simulink model "controlMDLV2"  (Simulink 7.9)
settings: Solver=ode45  StartTime=0.0  StopTime=inf  RelTol=1e-3
libraries: dspmtrx3 x7, simulink x7, utility x1, dspsolvers x1
settings Model: Creator=jorhabib  LastModifiedBy=jorhabib

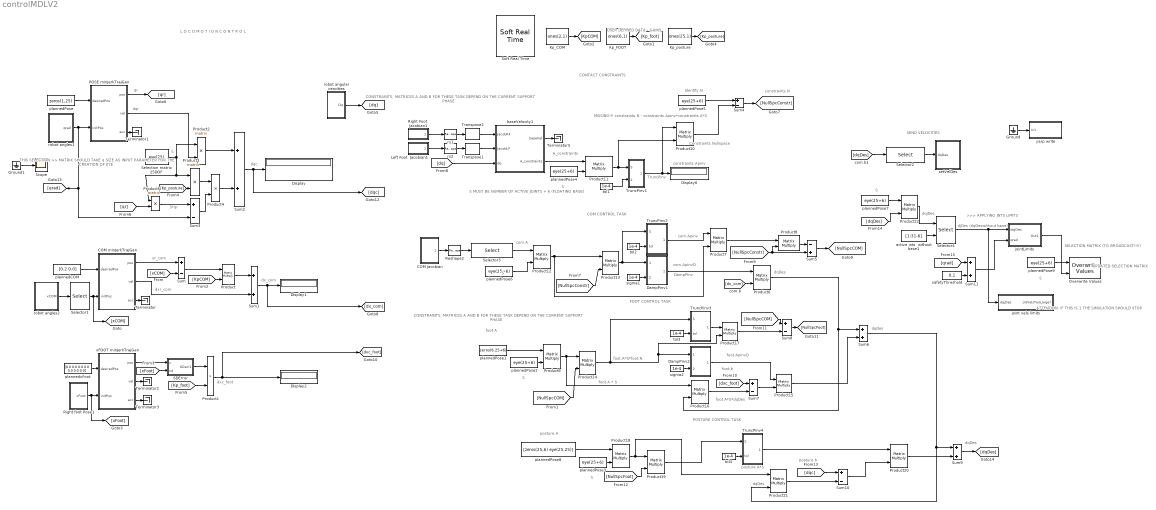
== system controlMDLV2 ==
  note: qr
  note: dqr
  note: S
  note: dqc
  note: S*qr
  note: THIS SELECTION    >>
      | MATRIX SHOULD
      | TAKE q SIZE AS
      | INPUT PARAMETER
      | FOR THE CREATION
      | OF EYE
  note: USER DEFINED DATA - GAINS
  note: xr_com
  note: dx_com
  note: dxr_com
  note: dxc_foot
  note: A_constraints
  note: S
  note: TruncPinv
  note: S MUST BE NUMBER OF
      | ACTIVE JOINTS
      | + 6 (FLOATING BASE)
  note: constraints.Apinv
  note: constraints.N
  note: Constraints
      | Nullspace
  note: MISSING!!! constraints.N - constraints.Apinv*constraints.A*S
  note: Identity.N
  note: CONTACT CONSTRAINTS
  note: CONSTRAINTS, MATRICES
      |  A AND B FOR THESE TASK DEPEND
      | ON THE CURRENT SUPPORT PHASE
  note: DampPInv
  note: com.A
  note: S
  note: com.ApinvD
  note: COM CONTROL TASK
  note: FOOT CONTROL TASK
  note: dqDes
  note: com.Apinv
  note: CONSTRAINTS, MATRICES
      |  A AND B FOR THESE TASK DEPEND
      | ON THE CURRENT SUPPORT PHASE
  note: S
  note: foot.A
  note: dqDes
  note: POSTURE CONTROL TASK
  note: posture.A
  note: S
  note: posture.A*S
  note: dqDes
  note: dqDes
  note: foot.ApinvD
  note: foot.b
  note: foot.A*S*dqDes
  note: posture.b
  note: foot.A * S
  note: foot.A*S*foot.N
  note: SEND VELOCITIES
  note: L O C O M O T I O N C O N T R O L
  note: S
  note: dqjDes
  note: >>> APPLYING JNTS LIMITS
  note: djDes
      |  (dqDeswithout base)
  note: SELECTION MATRIX
      |  (TO BROADCAST!!!!)
  note: S
  note: UPDATED
      | SELECTION
      | MATRIX
  note: ATTENTION: IF THIS IS 1
      | THE SIMULATION
      | SHOULD STOP
  6DError : Subsystem
  COM Jacobian : Subsystem
  COM minJerkTrajGen : Subsystem
  DampPinv1 : Subsystem  mask{tol=1e-4}
      mask prompts: tol "Tolerance"
  DampPinv2 : Subsystem  mask{tol=1e-4}
      mask prompts: tol "Tolerance"
  Display{,1..2,6} (4 alike) : Display
  Ground : Ground
  Ground1 : Ground
  Kp_COM : Constant  Value=ones(2,1)
  Kp_FOOT : Constant  Value=ones(6,1)
  Kp_posture : Constant  Value=ones(25,1)
  Left Foot  Jacobian1 : Subsystem
  Overwrite Values : dspmtrx3/Overwrite Values  OverWriteDiag=Submatrix  valFrom2ndIP=Second input port  ConstValue=0  RowSpan=Range of rows  RowStartMode=Index  RowStartIndex=7  RowEndMode=Last  RowEndIndex=31  ColSpan=Range of columns  ColStartMode=Index  ColStartIndex=7  ColEndMode=Last  ColEndIndex=1  DiagSpan=Range of elements  DiagStartMode=Index  DiagStartIndex=2  DiagEndMode=Index  DiagEndIndex=4
  POSE minJerkTrajGen : Subsystem
  Product{,2..3,5..22} (21 alike) : Product  Multiplication=Matrix(*)  RndMeth=Zero
  Product1 : Product  RndMeth=Zero
  Product4 : Product  RndMeth=Zero
  Reshape2 : Reshape  OutputDimensionality=Customize  OutputDimensions=[6,31]
  Right Foot  Jacobian1 : Subsystem
  Right foot Pose1 : Subsystem
  Scope : Scope
  Selection matrix 25DOF : Constant  Value=eye(25)
  Selector1 : Selector  IndexMode=Zero-based  InputPortWidth=7  IndexOptions=Index vector (dialog)  Indices=[0:1]  OutputSizes=1
  Selector2 : Selector  InputPortWidth=31  IndexOptions=Index vector (dialog)  Indices=[7:31]  OutputSizes=1
  Selector3 : Selector  NumberOfDimensions=2  IndexMode=Zero-based  InputPortWidth=7  IndexOptions=Starting index (dialog),Starting index (dialog)  Indices=0,0  OutputSizes=2,25+6
  Selector4 : Selector  InputPortWidth=31  IndexOptions=Index vector (port)  Indices=[0:1]  OutputSizes=1
  Soft Real Time : utility/Soft Real Time  x=0.050
  Sum{,3..4,7..8,10} (6 alike) : Sum  Inputs=+-
  Sum{1..2,6,9,11} (5 alike) : Sum
  Sum5 : Sum  Inputs=-+
  Terminator{,1..3,5} (5 alike) : Terminator
  Transpose1 : dspmtrx3/Transpose  Hermitian=off  overflowFlag=off
  Transpose2 : dspmtrx3/Transpose  Hermitian=off  overflowFlag=off
  TruncPinv1 : Subsystem  mask{tol=1e-4}
      mask prompts: tol "Tolerance"
  TruncPinv2 : Subsystem  mask{tol=1e-4}
      mask prompts: tol "Tolerance"
  TruncPinv3 : Subsystem  mask{tol=1e-4}
      mask prompts: tol "Tolerance"
  TruncPinv4 : Subsystem  mask{tol=1e-4}
      mask prompts: tol "Tolerance"
  active jnts  without base1 : Constant  Value=[1:31-6]
  baseVelocity1 : Subsystem
  joint vels limits : Subsystem  mask{dqMax=1.0}
      mask prompts: dqMax "Maximum joint velocity"
      mask help:
      | Type a vector with the maximum values for each joint (e.g. 150*ones(25,1) for a 25 DOF robot)
      | Same for minimum joint limits.
      mask init:
      | qMax = 150*ones(25,1)
      | qMin = -150*ones(25,1)
      | thr = 0.1
  jointLimits : Subsystem  mask{qMax=150*ones(25,1), qMin=-150*ones(25,1), thr=0.1}
      mask prompts: qMax "Maximum joint angles vector"; qMin "Minimum joint angles vector"; thr "Threshold before hitting joint limit"
      mask help:
      | Type a vector with the maximum values for each joint (e.g. 150*ones(25,1) for a 25 DOF robot)
      | Same for minimum joint limits.
      mask init:
      | qMax = 150*ones(25,1)
      | qMin = -150*ones(25,1)
      | thr = 0.1
  plannedCOM : Constant  Value=[0.2 0.0]
  plannedPose : Constant  Value=zeros(1,25)
  plannedPose1 : Constant  Value=zeros(6,25+6)
  plannedPose{2..7,9} (7 alike) : Constant  Value=eye(25+6)
  plannedPose8 : Constant  Value=[zeros(25,6) eye(25,25)]
  plannedxFoot : Constant  Value=[0.0 0.0 0.0 0.0 0.0 0.0 0.0]
  robot angles1 : Subsystem
  robot angles2 : Subsystem
  robot angular veocities : Subsystem
  rs1 : Reshape  OutputDimensionality=Customize  OutputDimensions=[31,6]
  rs2 : Reshape  OutputDimensionality=Customize  OutputDimensions=[31,6]
  safetyThreshold : Constant  Value=0.1
  setVelDes : Subsystem
  sigma1 : Constant  Value=1e-4
  sigma2 : Constant  Value=1e-4
  tol{1..4} (4 alike) : Constant  Value=1e-4
  xFOOT minJerkTrajGen : Subsystem
  yarp write : Subsystem  mask{port_name='/ywrite:o'}
      mask prompts: port_name "Specify port name starting with "/" e.g. '/port/input:i'"
  wires:
  robot angles1/1(qrad) -> [qrad], Sum3/2, POSE minJerkTrajGen/2(initPos)
  plannedPose/1 -> POSE minJerkTrajGen/1(desiredPos)
  Selection matrix 25DOF/1 -> Product2/1, Product5/1, Product3/1
  Product2/1 -> Sum2/1
  [Kp_posture] -> Product3/2
  Product3/1 -> Product4/1
  Sum3/1 -> Product4/2
  Product4/1 -> Sum2/2
  Sum2/1 -> [dqc], Display/1
  Product5/1 -> Sum3/1
  POSE minJerkTrajGen/3(acc) -> Terminator1/1
  POSE minJerkTrajGen/1(pos) -> [qr]
  [qr] -> Product5/2
  POSE minJerkTrajGen/2(vel) -> Product2/2
  Kp_COM/1 -> [KpCOM]
  Kp_FOOT/1 -> [Kp_foot]
  Kp_posture/1 -> [Kp_posture]
  plannedCOM/1 -> COM minJerkTrajGen/1(desiredPos)
  COM minJerkTrajGen/1(pos) -> Sum/1
  COM minJerkTrajGen/3(acc) -> Terminator/1
  [xCOM] -> Sum/2
  Sum/1 -> Product/1
  [KpCOM] -> Product/2
  Product/1 -> Sum1/1
  COM minJerkTrajGen/2(vel) -> Sum1/2
  Sum1/1 -> [dx_com], Display1/1
  Selector1/1 -> [xCOM], COM minJerkTrajGen/2(initPos)
  robot angles2/1(xCOM) -> Selector1/1
  xFOOT minJerkTrajGen/1(pos) -> 6DError/1(x)
  Right foot Pose1/1(xFoot) -> [xFoot], xFOOT minJerkTrajGen/2(initPos)
  plannedxFoot/1 -> xFOOT minJerkTrajGen/1(desiredPos)
  [xFoot] -> 6DError/2(xd)
  [Kp_foot] -> Product1/2
  Product1/1 -> [dxc_foot], Display2/1
  6DError/1(6Derr1) -> Product1/1
  xFOOT minJerkTrajGen/3(acc) -> Terminator3/1
  xFOOT minJerkTrajGen/2(vel) -> Terminator2/1
  robot angular veocities/1(Dq) -> [dq]
  Right Foot  Jacobian1/1(Jacobian) -> rs1/1
  Left Foot  Jacobian1/1(Jacobian) -> rs2/1
  [dq] -> baseVelocity1/3(dq)
  baseVelocity1/2(A_constraints) -> Product11/1
  plannedPose4/1 -> Product11/2
  tol1/1 -> TruncPinv1/2(tol)
  Product11/1 -> TruncPinv1/1(S), Product10/2
  TruncPinv1/1(Tpinv) -> Display6/1, Product10/1
  baseVelocity1/1(baseVel) -> Terminator5/1
  Product10/1 -> Sum4/2
  plannedPose5/1 -> Sum4/1
  Sum4/1 -> [NullSpcConstr]
  sigma1/1 -> DampPinv1/2(sigma)
  DampPinv1/1(DPinv) -> Product6/1
  COM Jacobian/1(Jacobian) -> Reshape2/1
  Reshape2/1 -> Selector3/1
  Selector3/1 -> Product12/1
  plannedPose6/1 -> Product12/2
  Product12/1 -> Product7/2, Product13/1
  [NullSpcConstr] -> Product13/2
  Product13/1 -> DampPinv1/1(mat), TruncPinv2/1(S)
  [dx_com] -> Product6/2
  Product6/1 -> Product16/2, Sum6/1
  tol2/1 -> TruncPinv2/2(tol)
  TruncPinv2/1(Tpinv) -> Product7/1
  Product7/1 -> Product8/1
  [NullSpcConstr] -> Sum5/2, Product8/2
  Product8/1 -> Sum5/1
  Sum5/1 -> [NullSpcCOM]
  tol3/1 -> TruncPinv3/2(tol)
  sigma2/1 -> DampPinv2/2(sigma)
  plannedPose1/1 -> Product9/1
  plannedPose2/1 -> Product9/2
  Product9/1 -> Product16/1, Product14/1
  [NullSpcCOM] -> Product14/2
  Product14/1 -> Product17/2, DampPinv2/1(mat), TruncPinv3/1(S)
  [dxc_foot] -> Sum7/1
  Product16/1 -> Sum7/2
  Product15/1 -> Sum6/2
  [NullSpcCOM] -> Sum8/1
  TruncPinv3/1(Tpinv) -> Product17/1
  Product17/1 -> Sum8/2
  Sum8/1 -> [NullSpcFoot]
  tol4/1 -> TruncPinv4/2(tol)
  plannedPose3/1 -> Product18/2
  plannedPose8/1 -> Product18/1
  Product18/1 -> Product21/1, Product19/1
  [NullSpcFoot] -> Product19/2
  Product19/1 -> TruncPinv4/1(S)
  Sum6/1 -> Product21/2, Sum9/1
  TruncPinv4/1(Tpinv) -> Product20/1
  [dqc] -> Sum10/1
  Product21/1 -> Sum10/2
  Sum10/1 -> Product20/2
  Product20/1 -> Sum9/2
  DampPinv2/1(DPinv) -> Product15/1
  Sum7/1 -> Product15/2
  Sum9/1 -> [dqDes]
  rs1/1 -> Transpose2/1
  rs2/1 -> Transpose1/1
  Transpose2/1 -> baseVelocity1/1(JacobRF)
  Transpose1/1 -> baseVelocity1/2(JacobLF)
  [dqDes] -> Selector2/1
  Selector2/1 -> setVelDes/1(dqDes)
  plannedPose7/1 -> Product22/1
  [dqDes] -> Product22/2
  Product22/1 -> Selector4/1
  active jnts  without base1/1 -> Selector4/2
  Selector4/1 -> jointLimits/1(dqjDes), joint vels limits/1(dqjDes)
  Sum11/1 -> jointLimits/2(qrad)
  [qrad] -> Sum11/1
  safetyThreshold/1 -> Sum11/2
  plannedPose9/1 -> Overwrite Values/1
  jointLimits/1(Out1) -> Overwrite Values/2
  Ground/1 -> yarp write/1(In1)
  Ground1/1 -> Scope/1

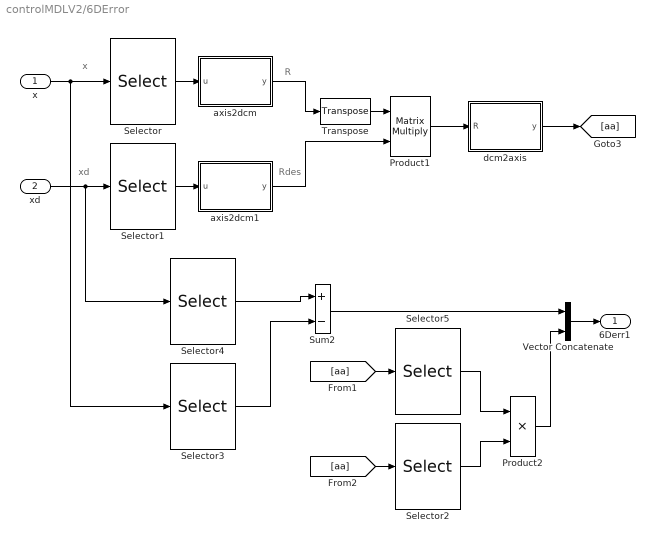
== system controlMDLV2/6DError ==
  note: xd
  note: x
  note: Rdes
  note: R
  x : Inport
  xd : Inport  Port=2
  Product1 : Product  Multiplication=Matrix(*)  RndMeth=Zero
  Product2 : Product  RndMeth=Zero
  Selector : Selector  IndexMode=Zero-based  InputPortWidth=7  IndexOptions=Index vector (dialog)  Indices=[3:6]  OutputSizes=1
  Selector1 : Selector  IndexMode=Zero-based  InputPortWidth=7  IndexOptions=Index vector (dialog)  Indices=[3:6]  OutputSizes=1
  Selector2 : Selector  IndexMode=Zero-based  InputPortWidth=4  IndexOptions=Index vector (dialog)  Indices=[0:2]  OutputSizes=1
  Selector3 : Selector  IndexMode=Zero-based  InputPortWidth=7  IndexOptions=Index vector (dialog)  Indices=[0:2]  OutputSizes=1
  Selector4 : Selector  IndexMode=Zero-based  InputPortWidth=7  IndexOptions=Index vector (dialog)  Indices=[0:2]  OutputSizes=1
  Selector5 : Selector  IndexMode=Zero-based  InputPortWidth=4  IndexOptions=Index vector (dialog)  Indices=3  OutputSizes=1
  Sum2 : Sum  Inputs=+-
  Transpose : dspmtrx3/Transpose  Hermitian=off  overflowFlag=off
  Vector Concatenate : Concatenate
  axis2dcm : MATLAB Function  TreatAsAtomicUnit=on
  axis2dcm1 : MATLAB Function  TreatAsAtomicUnit=on
  dcm2axis : MATLAB Function  TreatAsAtomicUnit=on
  6Derr1 : Outport
  wires:
  dcm2axis/1(y) -> [aa]
  Sum2/1 -> Vector Concatenate/1
  Vector Concatenate/1 -> 6Derr1/1
  [aa] -> Selector5/1
  Product2/1 -> Vector Concatenate/2
  Selector2/1 -> Product2/2
  Selector5/1 -> Product2/1
  [aa] -> Selector2/1
  Selector3/1 -> Sum2/2
  Selector4/1 -> Sum2/1
  Product1/1 -> dcm2axis/1(R)
  axis2dcm1/1(y) -> Product1/2
  axis2dcm/1(y) -> Transpose/1
  Transpose/1 -> Product1/1
  xd/1 -> Selector4/1, Selector1/1
  x/1 -> Selector3/1, Selector/1
  Selector1/1 -> axis2dcm1/1(u)
  Selector/1 -> axis2dcm/1(u)

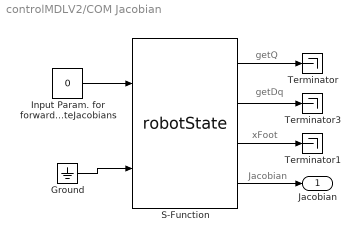
== system controlMDLV2/COM Jacobian ==
  note: getDq
  note: xFoot
  note: getQ
  note: Jacobian
  Ground : Ground
  "Input Param. for forwardKinematics and  computeJacobians " : Constant  Value=0  OutDataTypeStr=int8
  S-Function : S-Function  FunctionName=robotState  Parameters=val,robotname,localname  EnableBusSupport=off  mask{val=3, robotname='icubSim', localname='robotState'}
      mask prompts: val "Value"; robotname "Robot Name (icub - icubSim)"; localname "Module Name"
  Terminator : Terminator
  Terminator1 : Terminator
  Terminator3 : Terminator
  Jacobian : Outport
  wires:
  Ground/1 -> S-Function/2
  S-Function/2 -> Terminator3/1
  S-Function/1 -> Terminator/1
  S-Function/3 -> Terminator1/1
  "Input Param. for forwardKinematics and  computeJacobians "/1 -> S-Function/1
  S-Function/4 -> Jacobian/1

== system controlMDLV2/COM minJerkTrajGen ==
  desiredPos : Inport
  initPos : Inport  Port=2
  S-Function : S-Function  FunctionName=minJerkGenerator  Parameters=dim, rate, tt  EnableBusSupport=off  mask{dim=2, rate=10, tt=4}
      mask prompts: dim "Trajectory dimension (int)"; rate "Simulation rate (int) [ms]"; tt "Trajectory time [s]"
  pos : Outport
  vel : Outport  Port=2
  acc : Outport  Port=3
  wires:
  S-Function/2 -> vel/1
  S-Function/1 -> pos/1
  S-Function/3 -> acc/1
  initPos/1 -> S-Function/1
  desiredPos/1 -> S-Function/2

== system controlMDLV2/DampPinv1 ==
  mat : Inport
  sigma : Inport  Port=2
  Damped Pseudo Inverse : MATLAB Function  TreatAsAtomicUnit=on
  DPinv : Outport
  wires:
  sigma/1 -> Damped Pseudo Inverse/2(sigma)
  Damped Pseudo Inverse/1(DPinv) -> DPinv/1
  mat/1 -> Damped Pseudo Inverse/1(mat)

== system controlMDLV2/DampPinv2 ==
  mat : Inport
  sigma : Inport  Port=2
  Damped Pseudo Inverse : MATLAB Function  TreatAsAtomicUnit=on
  DPinv : Outport
  wires:
  mat/1 -> Damped Pseudo Inverse/1(mat)
  Damped Pseudo Inverse/1(DPinv) -> DPinv/1
  sigma/1 -> Damped Pseudo Inverse/2(sigma)

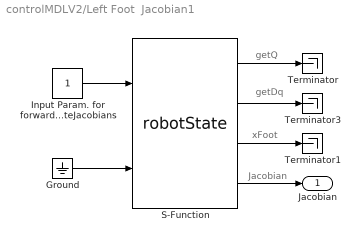
== system controlMDLV2/Left Foot  Jacobian1 ==
  note: Jacobian
  note: getQ
  note: xFoot
  note: getDq
  Ground : Ground
  "Input Param. for forwardKinematics and  computeJacobians " : Constant  OutDataTypeStr=int8
  S-Function : S-Function  FunctionName=robotState  Parameters=val,robotname,localname  EnableBusSupport=off  mask{val=3, robotname='icubSim', localname='robotState'}
      mask prompts: val "Value"; robotname "Robot Name (icub - icubSim)"; localname "Module Name"
  Terminator : Terminator
  Terminator1 : Terminator
  Terminator3 : Terminator
  Jacobian : Outport
  wires:
  S-Function/4 -> Jacobian/1
  "Input Param. for forwardKinematics and  computeJacobians "/1 -> S-Function/1
  S-Function/3 -> Terminator1/1
  S-Function/1 -> Terminator/1
  S-Function/2 -> Terminator3/1
  Ground/1 -> S-Function/2

== system controlMDLV2/POSE minJerkTrajGen ==
  desiredPos : Inport
  initPos : Inport  Port=2
  S-Function : S-Function  FunctionName=minJerkGenerator  Parameters=dim, rate, tt  EnableBusSupport=off  mask{dim=25, rate=10, tt=4}
      mask prompts: dim "Trajectory dimension (int)"; rate "Simulation rate (int) [ms]"; tt "Trajectory time [s]"
  pos : Outport
  vel : Outport  Port=2
  acc : Outport  Port=3
  wires:
  desiredPos/1 -> S-Function/2
  initPos/1 -> S-Function/1
  S-Function/3 -> acc/1
  S-Function/1 -> pos/1
  S-Function/2 -> vel/1

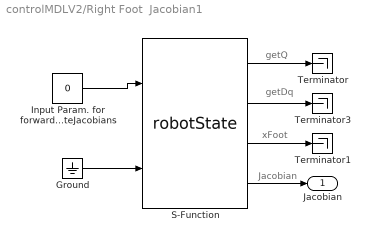
== system controlMDLV2/Right Foot  Jacobian1 ==
  note: getDq
  note: xFoot
  note: getQ
  note: Jacobian
  Ground : Ground
  "Input Param. for forwardKinematics and  computeJacobians " : Constant  Value=0  OutDataTypeStr=int8
  S-Function : S-Function  FunctionName=robotState  Parameters=val,robotname,localname  EnableBusSupport=off  mask{val=3, robotname='icubSim', localname='robotState'}
      mask prompts: val "Value"; robotname "Robot Name (icub - icubSim)"; localname "Module Name"
  Terminator : Terminator
  Terminator1 : Terminator
  Terminator3 : Terminator
  Jacobian : Outport
  wires:
  S-Function/2 -> Terminator3/1
  S-Function/1 -> Terminator/1
  S-Function/3 -> Terminator1/1
  "Input Param. for forwardKinematics and  computeJacobians "/1 -> S-Function/1
  S-Function/4 -> Jacobian/1
  Ground/1 -> S-Function/2

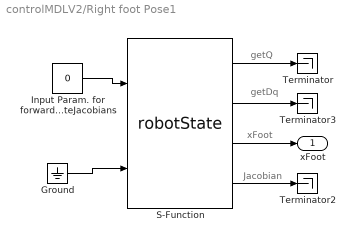
== system controlMDLV2/Right foot Pose1 ==
  note: Jacobian
  note: getQ
  note: xFoot
  note: getDq
  Ground : Ground
  "Input Param. for forwardKinematics and  computeJacobians " : Constant  Value=0  OutDataTypeStr=int8
  S-Function : S-Function  FunctionName=robotState  Parameters=val,robotname,localname  EnableBusSupport=off  mask{val=2, robotname='icubSim', localname='robotState'}
      mask prompts: val "Value"; robotname "Robot Name (icub - icubSim)"; localname "Module Name"
  Terminator : Terminator
  Terminator2 : Terminator
  Terminator3 : Terminator
  xFoot : Outport
  wires:
  Ground/1 -> S-Function/2
  S-Function/4 -> Terminator2/1
  "Input Param. for forwardKinematics and  computeJacobians "/1 -> S-Function/1
  S-Function/3 -> xFoot/1
  S-Function/1 -> Terminator/1
  S-Function/2 -> Terminator3/1

== system controlMDLV2/TruncPinv1 ==
  S : Inport
  tol : Inport  Port=2
  Truncated PseudoInverse : MATLAB Function  TreatAsAtomicUnit=on
  Tpinv : Outport
  wires:
  S/1 -> Truncated PseudoInverse/1(mat)
  Truncated PseudoInverse/1(TPinv) -> Tpinv/1
  tol/1 -> Truncated PseudoInverse/2(tol)

== system controlMDLV2/TruncPinv2 ==
  S : Inport
  tol : Inport  Port=2
  Truncated PseudoInverse : MATLAB Function  TreatAsAtomicUnit=on
  Tpinv : Outport
  wires:
  S/1 -> Truncated PseudoInverse/1(mat)
  Truncated PseudoInverse/1(TPinv) -> Tpinv/1
  tol/1 -> Truncated PseudoInverse/2(tol)

== system controlMDLV2/TruncPinv3 ==
  S : Inport
  tol : Inport  Port=2
  Truncated PseudoInverse : MATLAB Function  TreatAsAtomicUnit=on
  Tpinv : Outport
  wires:
  tol/1 -> Truncated PseudoInverse/2(tol)
  Truncated PseudoInverse/1(TPinv) -> Tpinv/1
  S/1 -> Truncated PseudoInverse/1(mat)

== system controlMDLV2/TruncPinv4 ==
  S : Inport
  tol : Inport  Port=2
  Truncated PseudoInverse : MATLAB Function  TreatAsAtomicUnit=on
  Tpinv : Outport
  wires:
  S/1 -> Truncated PseudoInverse/1(mat)
  Truncated PseudoInverse/1(TPinv) -> Tpinv/1
  tol/1 -> Truncated PseudoInverse/2(tol)

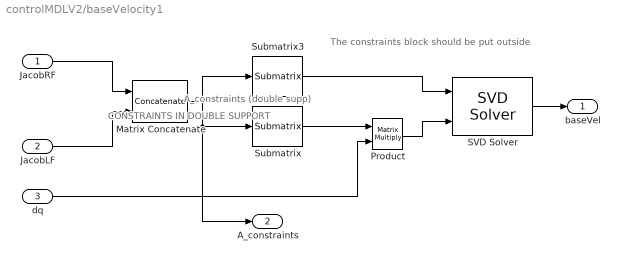
== system controlMDLV2/baseVelocity1 ==
  note: A_constraints
      | (double supp)
  note: CONSTRAINTS IN DOUBLE SUPPORT
  note: The constraints block should be put outside
  JacobRF : Inport
  JacobLF : Inport  Port=2
  dq : Inport  Port=3
  Matrix Concatenate : Concatenate  Mode=Multidimensional array
  Product : Product  Multiplication=Matrix(*)  RndMeth=Zero
  SVD Solver : dspsolvers/SVD Solver  wanterr=off
  Submatrix : dspmtrx3/Submatrix  RowSpan=Range of rows  RowStartMode=First  RowStartIndex=1  RowEndMode=Last  RowEndIndex=1  ColSpan=Range of columns  ColStartMode=Index  ColStartIndex=7  ColEndMode=Last  ColEndIndex=1
  Submatrix3 : dspmtrx3/Submatrix  RowSpan=Range of rows  RowStartMode=First  RowStartIndex=1  RowEndMode=Last  RowEndIndex=1  ColSpan=Range of columns  ColStartMode=First  ColStartIndex=7  ColEndMode=Index  ColEndIndex=6
  baseVel : Outport
  A_constraints : Outport  Port=2
  wires:
  dq/1 -> Product/2
  Product/1 -> SVD Solver/2
  Submatrix/1 -> Product/1
  JacobLF/1 -> Matrix Concatenate/2
  SVD Solver/1 -> baseVel/1
  JacobRF/1 -> Matrix Concatenate/1
  Submatrix3/1 -> SVD Solver/1
  Matrix Concatenate/1 -> Submatrix3/1, Submatrix/1, A_constraints/1

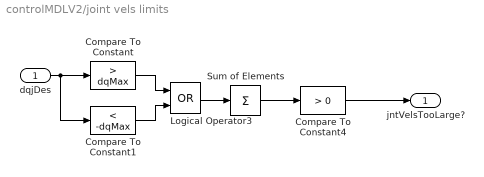
== system controlMDLV2/joint vels limits ==
  dqjDes : Inport
  Compare To Constant : simulink/Logic and Bit Operations/Compare To Constant  relop=>  const=dqMax  OutDataTypeStr=uint8
  Compare To Constant1 : simulink/Logic and Bit Operations/Compare To Constant  relop=<  const=-dqMax  OutDataTypeStr=uint8
  Compare To Constant4 : simulink/Logic and Bit Operations/Compare To Constant  relop=>  const=0  OutDataTypeStr=uint8
  Logical Operator3 : Logic  Operator=OR  AllPortsSameDT=off  OutDataTypeStr=boolean
  Sum of Elements : Sum  Inputs=+
  jntVelsTooLarge? : Outport
  wires:
  dqjDes/1 -> Compare To Constant/1, Compare To Constant1/1
  Compare To Constant/1 -> Logical Operator3/1
  Compare To Constant1/1 -> Logical Operator3/2
  Logical Operator3/1 -> Sum of Elements/1
  Sum of Elements/1 -> Compare To Constant4/1
  Compare To Constant4/1 -> jntVelsTooLarge?/1

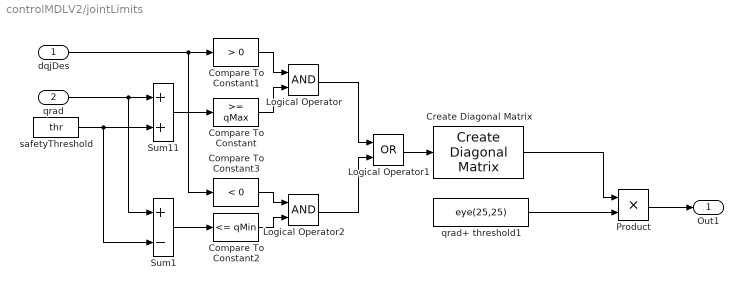
== system controlMDLV2/jointLimits ==
  dqjDes : Inport
  qrad : Inport  Port=2
  Compare To Constant : simulink/Logic and Bit Operations/Compare To Constant  relop=>=  const=qMax  OutDataTypeStr=uint8
  Compare To Constant1 : simulink/Logic and Bit Operations/Compare To Constant  relop=>  const=0  OutDataTypeStr=uint8
  Compare To Constant2 : simulink/Logic and Bit Operations/Compare To Constant  relop=<=  const=qMin  OutDataTypeStr=uint8
  Compare To Constant3 : simulink/Logic and Bit Operations/Compare To Constant  relop=<  const=0  OutDataTypeStr=uint8
  Create Diagonal Matrix : dspmtrx3/Create Diagonal Matrix
  Logical Operator : Logic  AllPortsSameDT=off  OutDataTypeStr=boolean
  Logical Operator1 : Logic  Operator=OR  AllPortsSameDT=off  OutDataTypeStr=boolean
  Logical Operator2 : Logic  AllPortsSameDT=off  OutDataTypeStr=boolean
  Product : Product  RndMeth=Zero
  Sum1 : Sum  Inputs=+-
  Sum11 : Sum
  qrad+ threshold1 : Constant  Value=eye(25,25)
  safetyThreshold : Constant  Value=thr
  Out1 : Outport
  wires:
  dqjDes/1 -> Compare To Constant1/1, Compare To Constant3/1
  qrad+ threshold1/1 -> Product/2
  Create Diagonal Matrix/1 -> Product/1
  Logical Operator/1 -> Logical Operator1/1
  Compare To Constant1/1 -> Logical Operator/1
  Compare To Constant/1 -> Logical Operator/2
  qrad/1 -> Sum11/1, Sum1/1
  safetyThreshold/1 -> Sum11/2, Sum1/2
  Sum11/1 -> Compare To Constant/1
  Logical Operator1/1 -> Create Diagonal Matrix/1
  Product/1 -> Out1/1
  Sum1/1 -> Compare To Constant2/1
  Compare To Constant2/1 -> Logical Operator2/2
  Compare To Constant3/1 -> Logical Operator2/1
  Logical Operator2/1 -> Logical Operator1/2

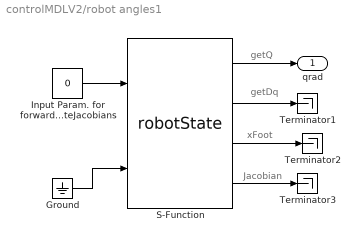
== system controlMDLV2/robot angles1 ==
  note: getDq
  note: xFoot
  note: getQ
  note: Jacobian
  Ground : Ground
  "Input Param. for forwardKinematics and  computeJacobians " : Constant  Value=0  OutDataTypeStr=int8
  S-Function : S-Function  FunctionName=robotState  Parameters=val,robotname,localname  EnableBusSupport=off  mask{val=0, robotname='icubSim', localname='robotState'}
      mask prompts: val "Value"; robotname "Robot Name (icub - icubSim)"; localname "Module Name"
  Terminator1 : Terminator
  Terminator2 : Terminator
  Terminator3 : Terminator
  qrad : Outport
  wires:
  Ground/1 -> S-Function/2
  S-Function/2 -> Terminator1/1
  S-Function/1 -> qrad/1
  S-Function/3 -> Terminator2/1
  "Input Param. for forwardKinematics and  computeJacobians "/1 -> S-Function/1
  S-Function/4 -> Terminator3/1

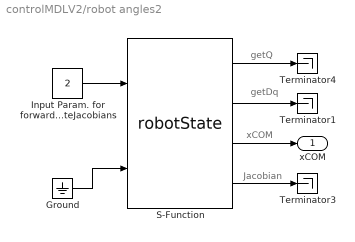
== system controlMDLV2/robot angles2 ==
  note: Jacobian
  note: getQ
  note: xCOM
  note: getDq
  Ground : Ground
  "Input Param. for forwardKinematics and  computeJacobians " : Constant  Value=2  OutDataTypeStr=int8
  S-Function : S-Function  FunctionName=robotState  Parameters=val,robotname,localname  EnableBusSupport=off  mask{val=2, robotname='icubSim', localname='robotState'}
      mask prompts: val "Value"; robotname "Robot Name (icub - icubSim)"; localname "Module Name"
  Terminator1 : Terminator
  Terminator3 : Terminator
  Terminator4 : Terminator
  xCOM : Outport
  wires:
  S-Function/4 -> Terminator3/1
  "Input Param. for forwardKinematics and  computeJacobians "/1 -> S-Function/1
  S-Function/3 -> xCOM/1
  S-Function/1 -> Terminator4/1
  S-Function/2 -> Terminator1/1
  Ground/1 -> S-Function/2

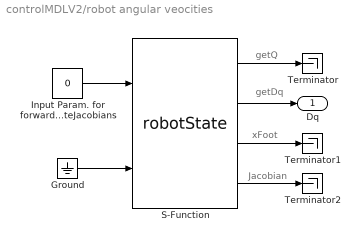
== system controlMDLV2/robot angular veocities ==
  note: getDq
  note: xFoot
  note: getQ
  note: Jacobian
  Ground : Ground
  "Input Param. for forwardKinematics and  computeJacobians " : Constant  Value=0  OutDataTypeStr=int8
  S-Function : S-Function  FunctionName=robotState  Parameters=val,robotname,localname  EnableBusSupport=off  mask{val=1, robotname='icubSim', localname='robotState'}
      mask prompts: val "Value"; robotname "Robot Name (icub - icubSim)"; localname "Module Name"
  Terminator : Terminator
  Terminator1 : Terminator
  Terminator2 : Terminator
  Dq : Outport
  wires:
  Ground/1 -> S-Function/2
  S-Function/2 -> Dq/1
  S-Function/1 -> Terminator/1
  S-Function/3 -> Terminator1/1
  "Input Param. for forwardKinematics and  computeJacobians "/1 -> S-Function/1
  S-Function/4 -> Terminator2/1

== system controlMDLV2/setVelDes ==
  note: Jacobian
  note: getQ
  note: xFoot
  note: getDq
  dqDes : Inport
  "Input Param. for forwardKinematics and  computeJacobians " : Constant  Value=0  OutDataTypeStr=int8
  S-Function : S-Function  FunctionName=robotState  Parameters=val,robotname,localname  EnableBusSupport=off  mask{val=4, robotname='icubSim', localname='robotState'}
      mask prompts: val "Value"; robotname "Robot Name (icub - icubSim)"; localname "Module Name"
  Terminator{1..4} (4 alike) : Terminator
  wires:
  S-Function/4 -> Terminator3/1
  "Input Param. for forwardKinematics and  computeJacobians "/1 -> S-Function/1
  S-Function/3 -> Terminator2/1
  S-Function/1 -> Terminator4/1
  S-Function/2 -> Terminator1/1
  dqDes/1 -> S-Function/2

== system controlMDLV2/xFOOT minJerkTrajGen ==
  desiredPos : Inport
  initPos : Inport  Port=2
  S-Function : S-Function  FunctionName=minJerkGenerator  Parameters=dim, rate, tt  EnableBusSupport=off  mask{dim=7, rate=10, tt=4}
      mask prompts: dim "Trajectory dimension (int)"; rate "Simulation rate (int) [ms]"; tt "Trajectory time [s]"
  pos : Outport
  vel : Outport  Port=2
  acc : Outport  Port=3
  wires:
  desiredPos/1 -> S-Function/2
  initPos/1 -> S-Function/1
  S-Function/3 -> acc/1
  S-Function/1 -> pos/1
  S-Function/2 -> vel/1

== system controlMDLV2/yarp write ==
  In1 : Inport
  S-Function : S-Function  FunctionName=yWrite  Parameters=port_name  EnableBusSupport=off
  wires:
  In1/1 -> S-Function/1

== matlab function 6DError/axis2dcm1 ==
  data: u input double; y output double
function y = fcn(u)
%#codegen

if length(u)<4
    y = 0;
else
    R = eye(4,4);
    theta = u(3+1);
    if theta == 0
        y = R;
    else
        v = zeros(3,1);
        c = cos(theta);
        s = sin(theta);
        C = 1 - c;
        
        xs = v(0+1)*s;
        ys = v(1+1)*s;
        zs = v(2+1)*s;
        xC = v(0+1)*C;
        yC = v(1+1)*C;
        zC = v(2+1)*C;
        xyC= v(0+1)*yC;
        yzC= v(1+1)*zC;
        zxC= v(2+1)*xC;
        
        R(0+1,0+1)=v(0+1)*xC+c;
        R(0+1,1+1)=xyC-zs;
        R(0+1,2+1)=zxC+ys;
        R(1+1,0+1)=xyC+zs;
        R(1+1,1+1)=v(1+1)*yC+c;
        R(1+1,2+1)=yzC-xs;
        R(2+1,0+1)=zxC-ys;
        R(2+1,1+1)=yzC+xs;
        R(2+1,2+1)=v(2+1)*zC+c;
        
        y = R;
    end
end

== matlab function 6DError/axis2dcm ==
  data: u input double; y output double
function y = fcn(u)
%#codegen

if length(u)<4
    y = 0;
else
    R = eye(4,4);
    theta = u(3+1);
    if theta == 0
        y = R;
    else
        v = zeros(3,1);
        c = cos(theta);
        s = sin(theta);
        C = 1 - c;
        
        xs = v(0+1)*s;
        ys = v(1+1)*s;
        zs = v(2+1)*s;
        xC = v(0+1)*C;
        yC = v(1+1)*C;
        zC = v(2+1)*C;
        xyC= v(0+1)*yC;
        yzC= v(1+1)*zC;
        zxC= v(2+1)*xC;
        
        R(0+1,0+1)=v(0+1)*xC+c;
        R(0+1,1+1)=xyC-zs;
        R(0+1,2+1)=zxC+ys;
        R(1+1,0+1)=xyC+zs;
        R(1+1,1+1)=v(1+1)*yC+c;
        R(1+1,2+1)=yzC-xs;
        R(2+1,0+1)=zxC-ys;
        R(2+1,1+1)=yzC+xs;
        R(2+1,2+1)=v(2+1)*zC+c;
        
        y = R;
    end
end

== matlab function 6DError/dcm2axis ==
  data: R input double; y output double
function y = fcn(R)
%#codegen

if size(R,1)<3 || size(R,2)<3
    y = zeros(4,1);
else
    v = zeros(4,1);
    v(0+1) = R(2+1,1+1) - R(1+1,2+1);
    v(1+1) = R(0+1,2+1) - R(2+1,0+1);
    v(2+1) = R(1+1,0+1) - R(0+1,1+1);
    v(3+1) = 0.0;
    
    r = norm(v);
    theta = atan2(0.5*r, 0.5*(R(0+1,0+1) + R(1+1,1+1) + R(2+1,2+1) - 1));
    
    if r<1e-9
        A = R(0+1:2+1, 0+1:2+1);
        [U,S,V] = svd(A - eye(3,3));
        
        v(0+1) = V(0+1,2+1);
        v(1+1) = V(1+1,2+1);
        v(2+1) = V(2+1,2+1);
        
        r = norm(v);
    end
    v = (1/r)*v;
    v(3+1) = theta;
    y = v;
end

end

== matlab function TruncPinv2/Truncated PseudoInverse ==
  data: mat input double; TPinv output double; tol input double
function TPinv  = fcn(mat,tol)
%#codegen
[U,S,V] = svd(mat,'econ');
% Setting to zero value
% Setting to 1/S(i,i) singular values greater than tol
 S(S>tol)=1./S(S>tol);
TPinv = V*pinv(S)*U';

== matlab function DampPinv2/Damped Pseudo Inverse ==
  data: mat input double; DPinv output double; sigma input double
function DPinv  = fcn(mat,sigma)
% Economody size svd of mat
[U,S,V] = svd(mat,'econ');
% Damped version of S with sigma
S(S>sigma)=S(S>sigma)./((S(S>sigma)).^2+sigma^2);
% Damped pseudoinverse
DPinv = V*pinv(S)*U';

== matlab function DampPinv1/Damped Pseudo Inverse ==
  data: mat input double; DPinv output double; sigma input double
function DPinv  = fcn(mat,sigma)
% Economody size svd of mat
[U,S,V] = svd(mat,'econ');
% Damped version of S with sigma
S(S>sigma)=S(S>sigma)./((S(S>sigma)).^2+sigma^2);
% Damped pseudoinverse
DPinv = V*pinv(S)*U';

== matlab function TruncPinv1/Truncated PseudoInverse ==
  data: mat input double; TPinv output double; tol input double
function TPinv  = fcn(mat,tol)
%#codegen
[U,S,V] = svd(mat,'econ');
% Setting to zero value
% Setting to 1/S(i,i) singular values greater than tol
 S(S>tol)=1./S(S>tol);
 TPinv = V*pinv(S)*U';

== matlab function TruncPinv3/Truncated PseudoInverse ==
  data: mat input double; TPinv output double; tol input double
function TPinv  = fcn(mat,tol)
%#codegen
[U,S,V] = svd(mat,'econ');
% Setting to zero value
% Setting to 1/S(i,i) singular values greater than tol
 S(S>tol)=1./S(S>tol);
TPinv = V*pinv(S)*U';

== matlab function TruncPinv4/Truncated PseudoInverse ==
  data: mat input double; TPinv output double; tol input double
function TPinv  = fcn(mat,tol)
%#codegen
[U,S,V] = svd(mat,'econ');
% Setting to 1/S(i,i) singular values greater than tol
 S(S>tol)=1./S(S>tol);
TPinv = V*pinv(S)*U';
